simulink model "Simple_battery_management_system"  (R2024b)
settings: Solver=VariableStepAuto  StartTime=0.0  StopTime=inf  RelTol=1e-3
settings Model: Creator=rohan  LastModifiedBy=rohan

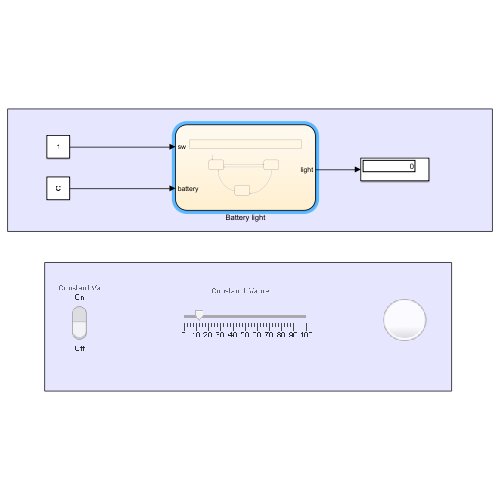
[thumbnail: Simulink's stored preview of the top-level diagram]
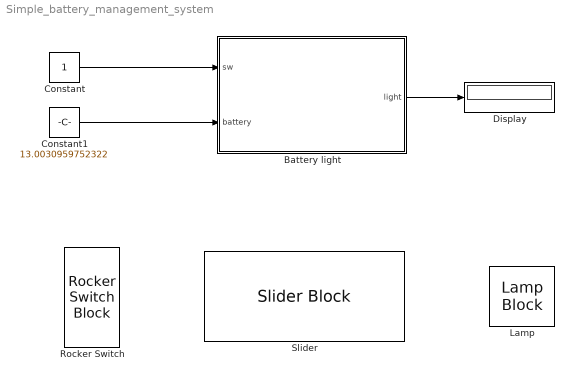
== system Simple_battery_management_system ==
  Battery light : Stateflow chart  TreatAsAtomicUnit=on
  Constant : Constant
  Constant1 : Constant  Value=13.0030959752322
  Display : Display
  Lamp : LampBlock  LabelPosition=Hide
  Rocker Switch : RockerSwitchBlock
      settings: Values={{'Off', 'On'}, [0 1]}
  Slider : SliderBlock
  wires:
  Constant1/1 -> Battery light/2(battery)
  Constant/1 -> Battery light/1(sw)
  Battery light/1(light) -> Display/1

== stateflow chart Simple_battery_management_system/Battery light ==
  state %Here, we have a simple battery management system for a light, we can see that when the battery (depicted using a slider in [group]
    this case) is less than 20% the FSM moves to  the low_battery state and the light color changes before turning completely off
    alerting the user that the battery is low.
  state OFF
    entry:
    light=0;
  state ON
    light=1;
  state LOW_Battery
    light=2;
  (default) -> OFF
  OFF -> ON : [sw==1 && battery>=20]
  ON -> OFF [order 2] : [sw==0]
  LOW_Battery -> OFF : after(5,sec)
  ON -> LOW_Battery [order 1] : [battery<20]
  data: sw input; battery input; light output
